simulink model "v1"  (R2017a)
settings: Solver=VariableStepAuto  StartTime=0.0  StopTime=240  RelTol=1e-3
libraries: fl_lib x18, nesl_utility x9
settings Model: Creator=mcall  LastModifiedBy=mcall
settings DataIOCC: SaveState=on  InspectSignalLogs=on

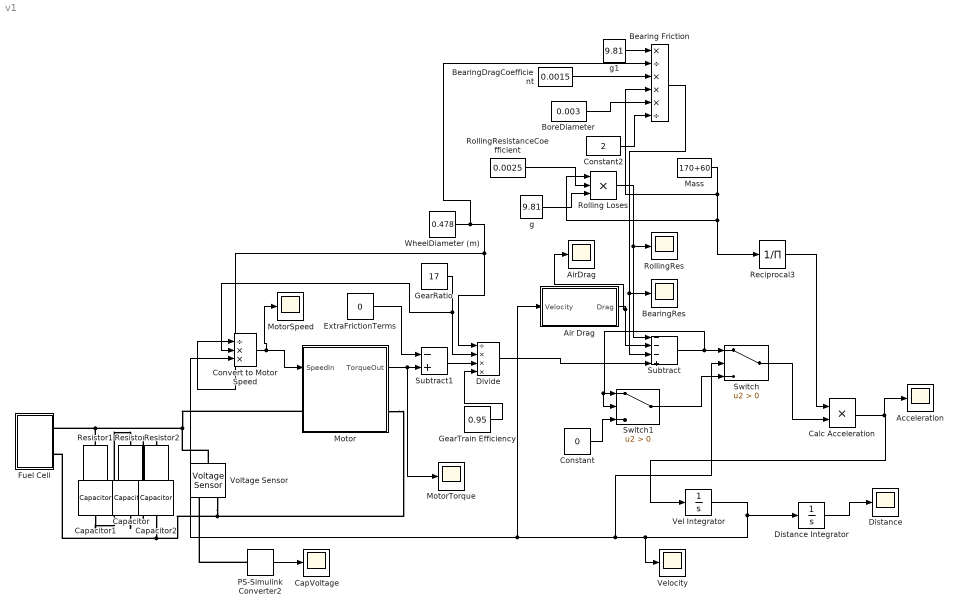
== system v1 ==
  Acceleration : Scope
  Air Drag : Subsystem
  AirDrag : Scope
  Bearing Friction : Product  Inputs=*/***/
  BearingDragCoefficient : Constant  Value=0.0015
  BearingRes : Scope
  BoreDiameter : Constant  Value=0.003
  Calc Acceleration : Product
  CapVoltage : Scope
  Capacitor : fl_lib/Electrical/Electrical Elements/Capacitor  c=58 F  r=1e-6 Ohm  g=0 1/Ohm  i_specify=off  i_priority=None  i=0 A  i_nominal_specify=off  i_nominal_unit=A  i_nominal_value=1  v_specify=on  v_priority=None  v=10 V  v_nominal_specify=off  v_nominal_unit=V  v_nominal_value=1  vc_specify=on  vc_priority=High  vc=10 V  vc_nominal_specify=off  vc_nominal_unit=V  vc_nominal_value=1
  Capacitor1 : fl_lib/Electrical/Electrical Elements/Capacitor  c=58 F  r=1e-6 Ohm  g=0 1/Ohm  i_specify=off  i_priority=None  i=0 A  i_nominal_specify=off  i_nominal_unit=A  i_nominal_value=1  v_specify=on  v_priority=None  v=10 V  v_nominal_specify=off  v_nominal_unit=V  v_nominal_value=1  vc_specify=on  vc_priority=High  vc=10 V  vc_nominal_specify=off  vc_nominal_unit=V  vc_nominal_value=1
  Capacitor2 : fl_lib/Electrical/Electrical Elements/Capacitor  c=58 F  r=1e-6 Ohm  g=0 1/Ohm  i_specify=off  i_priority=None  i=0 A  i_nominal_specify=off  i_nominal_unit=A  i_nominal_value=1  v_specify=on  v_priority=None  v=10 V  v_nominal_specify=off  v_nominal_unit=V  v_nominal_value=1  vc_specify=on  vc_priority=High  vc=10 V  vc_nominal_specify=off  vc_nominal_unit=V  vc_nominal_value=1
  Constant : Constant  Value=0
  Constant2 : Constant  Value=2
  Convert to Motor Speed : Product  Inputs=/**
  Distance : Scope
  Distance Integrator : Integrator
  Divide : Product  Inputs=/***
  ExtraFrictionTerms : Constant  Value=0
  Fuel Cell : Subsystem
  GearRatio : Constant  Value=17
  GearTrain Efficiency : Constant  Value=0.95
  Mass : Constant  Value=170+60
  Motor : Subsystem
  MotorSpeed : Scope
  MotorTorque : Scope
  PS-Simulink Converter2 : nesl_utility/PS-Simulink Converter  PhysicalDomain=network_engine_domain  SubClassName=ps_output  LeftPortType=input  RightPortType=output  PseudoPeriodic=off  Frequencies=[]  Unit=1  AffineConversion=off
  Reciprocal3 : Product  Inputs=/  SaturateOnIntegerOverflow=on  RndMeth=Zero
  Resistor : fl_lib/Electrical/Electrical Elements/Resistor  R=0.022 Ohm  i_specify=off  i_priority=None  i=0 A  i_nominal_specify=off  i_nominal_unit=A  i_nominal_value=1  v_specify=off  v_priority=None  v=0 V  v_nominal_specify=off  v_nominal_unit=V  v_nominal_value=1
  Resistor1 : fl_lib/Electrical/Electrical Elements/Resistor  R=0.022 Ohm  i_specify=off  i_priority=None  i=0 A  i_nominal_specify=off  i_nominal_unit=A  i_nominal_value=1  v_specify=off  v_priority=None  v=0 V  v_nominal_specify=off  v_nominal_unit=V  v_nominal_value=1
  Resistor2 : fl_lib/Electrical/Electrical Elements/Resistor  R=0.022 Ohm  i_specify=off  i_priority=None  i=0 A  i_nominal_specify=off  i_nominal_unit=A  i_nominal_value=1  v_specify=off  v_priority=None  v=0 V  v_nominal_specify=off  v_nominal_unit=V  v_nominal_value=1
  Rolling Loses : Product  Inputs=***
  RollingRes : Scope
  RollingResistanceCoefficient : Constant  Value=0.0025
  Subtract : Sum  Inputs=---+
  Subtract1 : Sum  Inputs=-+
  Switch : Switch  Criteria=u2 > Threshold
  Switch1 : Switch  Criteria=u2 > Threshold
  Vel Integrator : Integrator
  Velocity : Scope
  Voltage Sensor : fl_lib/Electrical/Electrical Sensors/Voltage Sensor
  WheelDiameter (m) : Constant  Value=0.478
  g : Constant  Value=9.81
  g1 : Constant  Value=9.81
  wires:
  Reciprocal3/1 -> Calc Acceleration/1
  Distance Integrator/1 -> Distance/1
  Motor/1(TorqueOut) -> MotorTorque/1, Subtract1/2
  ExtraFrictionTerms/1 -> Subtract1/1
  Subtract1/1 -> Divide/3
  GearTrain Efficiency/1 -> Divide/4
  GearRatio/1 -> Convert to Motor Speed/2, Divide/2
  WheelDiameter (m)/1 -> Bearing Friction/2, Divide/1, Convert to Motor Speed/1
  RollingResistanceCoefficient/1 -> Rolling Loses/2
  g/1 -> Rolling Loses/3
  Mass/1 -> Bearing Friction/4, Reciprocal3/1, Rolling Loses/1
  Rolling Loses/1 -> RollingRes/1, Subtract/1
  Air Drag/1(Drag) -> AirDrag/1, Subtract/2
  Convert to Motor Speed/1 -> MotorSpeed/1, Motor/1(SpeedIn)
  Calc Acceleration/1 -> Acceleration/1, Vel Integrator/1
  Vel Integrator/1 -> Velocity/1, Switch/2, Air Drag/1(Velocity), Convert to Motor Speed/3, Distance Integrator/1
  Subtract/1 -> Switch1/2, Switch1/1, Switch/1
  Switch/1 -> Calc Acceleration/2
  Switch1/1 -> Switch/3
  Constant/1 -> Switch1/3
  PS-Simulink Converter2/1 -> CapVoltage/1
  Divide/1 -> Subtract/4
  Bearing Friction/1 -> BearingRes/1, Subtract/3
  Constant2/1 -> Bearing Friction/6
  BoreDiameter/1 -> Bearing Friction/5
  BearingDragCoefficient/1 -> Bearing Friction/3
  g1/1 -> Bearing Friction/1
  connections:
  Motor/RConn1 -- Voltage Sensor/RConn2 -- Capacitor2/RConn1 -- Fuel Cell/RConn2
  Motor/LConn1 -- Voltage Sensor/LConn1 -- Resistor1/LConn1 -- Fuel Cell/RConn1
  PS-Simulink Converter2/LConn1 -- Voltage Sensor/RConn1
  Capacitor/LConn1 -- Resistor/RConn1
  Resistor1/RConn1 -- Capacitor1/LConn1
  Capacitor1/RConn1 -- Resistor/LConn1
  Capacitor/RConn1 -- Resistor2/LConn1
  Capacitor2/LConn1 -- Resistor2/RConn1

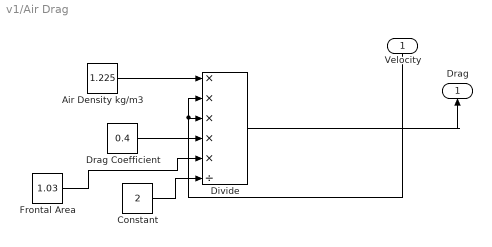
== system v1/Air Drag ==
  Velocity : Inport
  Air Density kg/m3 : Constant  Value=1.225
  Constant : Constant  Value=2
  Divide : Product  Inputs=*****/
  Drag Coefficient : Constant  Value=0.4
  Frontal Area : Constant  Value=1.03
  Drag : Outport
  wires:
  Divide/1 -> Drag/1
  Velocity/1 -> Divide/3, Divide/2
  Air Density kg/m3/1 -> Divide/1
  Frontal Area/1 -> Divide/5
  Drag Coefficient/1 -> Divide/4
  Constant/1 -> Divide/6

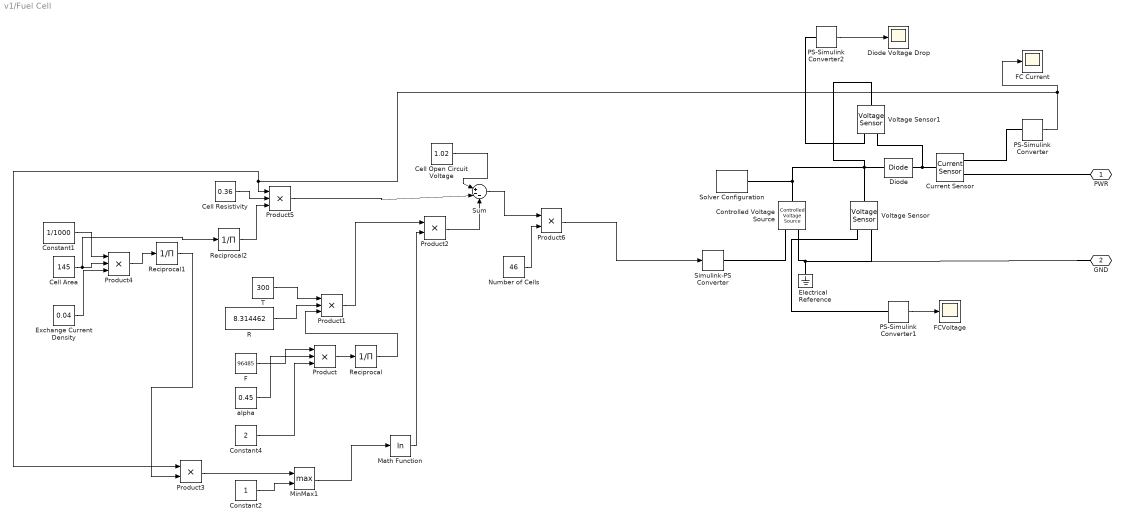
== system v1/Fuel Cell ==
  Cell Area : Constant  Value=145
  Cell Open Circuit Voltage : Constant  Value=1.02
  Cell Resistivity : Constant  Value=0.36
  Constant1 : Constant  Value=1/1000
  Constant2 : Constant
  Constant4 : Constant  Value=2
  Controlled Voltage Source : fl_lib/Electrical/Electrical Sources/Controlled Voltage Source
  Current Sensor : fl_lib/Electrical/Electrical Sensors/Current Sensor
  Diode : fl_lib/Electrical/Electrical Elements/Diode  Vf=0.6 V  Ron=0.3 Ohm  Goff=1e-8 1/Ohm  i_specify=off  i_priority=None  i=0 A  i_nominal_specify=off  i_nominal_unit=A  i_nominal_value=1  v_specify=off  v_priority=None  v=0 V  v_nominal_specify=off  v_nominal_unit=V  v_nominal_value=1
  Diode Voltage Drop : Scope
  Electrical Reference : fl_lib/Electrical/Electrical Elements/Electrical Reference
  Exchange Current Density : Constant  Value=0.04
  F : Constant  Value=96485
  FC Current : Scope
  FCVoltage : Scope
  Math Function : Math  Operator=log  SaturateOnIntegerOverflow=on
  MinMax1 : MinMax  Function=max  Inputs=2
  Number of Cells : Constant  Value=46
  PS-Simulink Converter : nesl_utility/PS-Simulink Converter  PhysicalDomain=network_engine_domain  SubClassName=ps_output  LeftPortType=input  RightPortType=output  PseudoPeriodic=off  Frequencies=[]  Unit=1  AffineConversion=off
  PS-Simulink Converter1 : nesl_utility/PS-Simulink Converter  PhysicalDomain=network_engine_domain  SubClassName=ps_output  LeftPortType=input  RightPortType=output  PseudoPeriodic=off  Frequencies=[]  Unit=1  AffineConversion=off
  PS-Simulink Converter2 : nesl_utility/PS-Simulink Converter  PhysicalDomain=network_engine_domain  SubClassName=ps_output  LeftPortType=input  RightPortType=output  PseudoPeriodic=off  Frequencies=[]  Unit=1  AffineConversion=off
  Product{,1,4..5} (4 alike) : Product  Inputs=3
  Product2 : Product
  Product3 : Product
  Product6 : Product
  R : Constant  Value=8.314462
  Reciprocal : Product  Inputs=/  SaturateOnIntegerOverflow=on  RndMeth=Zero
  Reciprocal1 : Product  Inputs=/  SaturateOnIntegerOverflow=on  RndMeth=Zero
  Reciprocal2 : Product  Inputs=/  SaturateOnIntegerOverflow=on  RndMeth=Zero
  Simulink-PS Converter : nesl_utility/Simulink-PS Converter  PhysicalDomain=network_engine_domain  SubClassName=ps_input  LeftPortType=input  RightPortType=output  PseudoPeriodic=off  Frequencies=[]  NoiseDistribution=none  NoiseParameters=[]  Unit=1  AffineConversion=off  FilteringAndDerivatives=provide  SimscapeFilterOrder=1  InputFilterTimeConstant=0.001  UdotUserProvided=0
  Solver Configuration : nesl_utility/Solver Configuration  PhysicalDomain=network_engine_domain  SubClassName=solver  LeftPortType=input  RightPortType=generic  Accelerate=off  Tones=[]  Harmonics=[]  SimulateNoise=off  Profile=off  UseLocalSampling=off  EnableSwitchedLinearOptims=on  FrequencyDomain=off  UseCCode=off  RelTol=0.001  AbsTol=1e-06  MinStep=1e-09  ToWorkspace=off  RevertToSquareIcSolve=off  NumHomotopyIterations=100  PhasorMode=off  PhasorModeNumHarmonics=1  OverrideAbsTol=off  DoDC=off  ResidualTolerance=1e-09  UseLocalSolver=off  LocalSolverChoice=NE_BACKWARD_EULER_ADVANCER  LocalSolverSampleTime=0.001  DoFixedCost=off  MaxNonlinIter=3  MaxModeIter=2  LinearAlgebra=Sparse  DelaysMemoryBudget=1024  AutomaticFiltering=on  FilteringTimeConstant=0.001
  Sum : Sum  Inputs=|+--
  T : Constant  Value=300
  Voltage Sensor : fl_lib/Electrical/Electrical Sensors/Voltage Sensor
  Voltage Sensor1 : fl_lib/Electrical/Electrical Sensors/Voltage Sensor
  alpha : Constant  Value=0.45
  PWR : PMIOPort  Port=1  Side=Right
  GND : PMIOPort  Port=2  Side=Right
  wires:
  Product2/1 -> Sum/3
  Sum/1 -> Product6/1
  Number of Cells/1 -> Product6/2
  Product1/1 -> Product2/1
  Cell Open Circuit Voltage/1 -> Sum/1
  Product4/1 -> Reciprocal1/1
  Math Function/1 -> Product2/2
  Exchange Current Density/1 -> Product4/3
  R/1 -> Product1/2
  T/1 -> Product1/1
  Constant1/1 -> Product4/1
  Product/1 -> Reciprocal/1
  Reciprocal/1 -> Product1/3
  Reciprocal1/1 -> Product3/2
  Reciprocal2/1 -> Product5/3
  alpha/1 -> Product/2
  Constant4/1 -> Product/3
  Product5/1 -> Sum/2
  Cell Resistivity/1 -> Product5/2
  PS-Simulink Converter/1 -> FC Current/1, Product3/1, Product5/1
  PS-Simulink Converter1/1 -> FCVoltage/1
  F/1 -> Product/1
  Cell Area/1 -> Reciprocal2/1, Product4/2
  MinMax1/1 -> Math Function/1
  Product3/1 -> MinMax1/1
  Product6/1 -> Simulink-PS Converter/1
  Constant2/1 -> MinMax1/2
  PS-Simulink Converter2/1 -> Diode Voltage Drop/1
  connections:
  Electrical Reference/LConn1 -- GND/RConn1 -- Voltage Sensor/RConn2 -- Controlled Voltage Source/RConn2
  PWR/RConn1 -- Current Sensor/RConn2
  Voltage Sensor/RConn1 -- PS-Simulink Converter1/LConn1
  Simulink-PS Converter/RConn1 -- Controlled Voltage Source/RConn1
  Diode/LConn1 -- Voltage Sensor1/LConn1 -- Solver Configuration/RConn1 -- Controlled Voltage Source/LConn1 -- Voltage Sensor/LConn1
  Current Sensor/LConn1 -- Voltage Sensor1/RConn2 -- Diode/RConn1
  Current Sensor/RConn1 -- PS-Simulink Converter/LConn1
  Voltage Sensor1/RConn1 -- PS-Simulink Converter2/LConn1

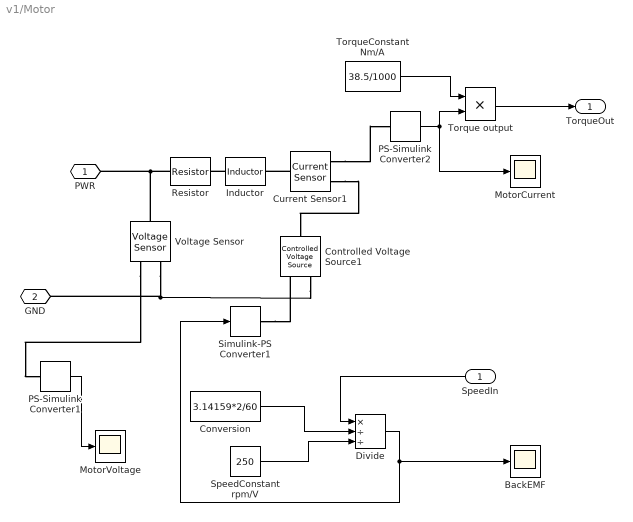
== system v1/Motor ==
  SpeedIn : Inport
  BackEMF : Scope
  Controlled Voltage Source1 : fl_lib/Electrical/Electrical Sources/Controlled Voltage Source
  Conversion : Constant  Value=3.14159*2/60
  Current Sensor1 : fl_lib/Electrical/Electrical Sensors/Current Sensor
  Divide : Product  Inputs=*//
  Inductor : fl_lib/Electrical/Electrical Elements/Inductor  l=0.072 mH  r=0 Ohm  g=1e-9 1/Ohm  i_specify=off  i_priority=None  i=0 A  i_nominal_specify=off  i_nominal_unit=A  i_nominal_value=1  v_specify=off  v_priority=None  v=0 V  v_nominal_specify=off  v_nominal_unit=V  v_nominal_value=1  i_L_specify=off  i_L_priority=High  i_L=0 A  i_L_nominal_specify=off  i_L_nominal_unit=A  i_L_nominal_value=1
  MotorCurrent : Scope
  MotorVoltage : Scope
  PS-Simulink Converter1 : nesl_utility/PS-Simulink Converter  PhysicalDomain=network_engine_domain  SubClassName=ps_output  LeftPortType=input  RightPortType=output  PseudoPeriodic=off  Frequencies=[]  Unit=1  AffineConversion=off
  PS-Simulink Converter2 : nesl_utility/PS-Simulink Converter  PhysicalDomain=network_engine_domain  SubClassName=ps_output  LeftPortType=input  RightPortType=output  PseudoPeriodic=off  Frequencies=[]  Unit=1  AffineConversion=off
  Resistor : fl_lib/Electrical/Electrical Elements/Resistor  R=1 Ohm  i_specify=off  i_priority=None  i=0 A  i_nominal_specify=off  i_nominal_unit=A  i_nominal_value=1  v_specify=off  v_priority=None  v=0 V  v_nominal_specify=off  v_nominal_unit=V  v_nominal_value=1
  Simulink-PS Converter1 : nesl_utility/Simulink-PS Converter  PhysicalDomain=network_engine_domain  SubClassName=ps_input  LeftPortType=input  RightPortType=output  PseudoPeriodic=off  Frequencies=[]  NoiseDistribution=none  NoiseParameters=[]  Unit=1  AffineConversion=off  FilteringAndDerivatives=provide  SimscapeFilterOrder=1  InputFilterTimeConstant=0.001  UdotUserProvided=0
  SpeedConstant rpm/V : Constant  Value=250
  Torque output : Product
  TorqueConstant Nm/A : Constant  Value=38.5/1000
  Voltage Sensor : fl_lib/Electrical/Electrical Sensors/Voltage Sensor
  PWR : PMIOPort  Port=1  Side=Left
  GND : PMIOPort  Port=2  Side=Right
  TorqueOut : Outport
  wires:
  PS-Simulink Converter2/1 -> MotorCurrent/1, Torque output/2
  Torque output/1 -> TorqueOut/1
  TorqueConstant Nm/A/1 -> Torque output/1
  SpeedIn/1 -> Divide/1
  SpeedConstant rpm/V/1 -> Divide/3
  Conversion/1 -> Divide/2
  PS-Simulink Converter1/1 -> MotorVoltage/1
  Divide/1 -> Simulink-PS Converter1/1, BackEMF/1
  connections:
  Current Sensor1/RConn2 -- Controlled Voltage Source1/LConn1
  Current Sensor1/LConn1 -- Inductor/RConn1
  Simulink-PS Converter1/RConn1 -- Controlled Voltage Source1/RConn1
  Current Sensor1/RConn1 -- PS-Simulink Converter2/LConn1
  Inductor/LConn1 -- Resistor/RConn1
  Resistor/LConn1 -- Voltage Sensor/LConn1 -- PWR/RConn1
  Controlled Voltage Source1/RConn2 -- Voltage Sensor/RConn2 -- GND/RConn1
  Voltage Sensor/RConn1 -- PS-Simulink Converter1/LConn1
